simulink model "state_space_verification"  (R2023a)
settings: Solver=ode45  StartTime=0.0  StopTime=5  RelTol=1e-3
InitFcn:
  | data = load("state_space.mat");
  | A = data.A;
  | B = data.B;
  | 
  | K = test();
libraries: simulink_extras x8
settings Model: Creator=Jason  LastModifiedBy=Jason

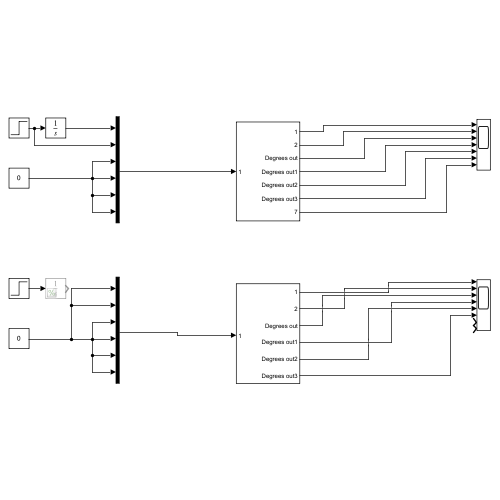
[thumbnail: Simulink's stored preview of the top-level diagram]
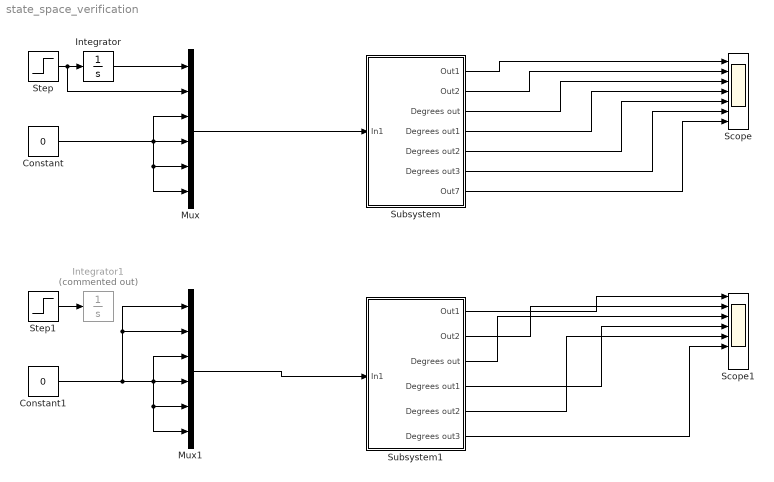
== system state_space_verification ==
  Constant : Constant  Value=0
  Constant1 : Constant  Value=0
  Integrator : Integrator
  Integrator1 : Integrator  Commented=on
  Mux : Mux  Inputs=6
  Mux1 : Mux  Inputs=6
  Scope : Scope  NumInputPorts=7
  Scope1 : Scope  NumInputPorts=8
  Step : Step  After=0.3  SampleTime=0
  Step1 : Step  SampleTime=0
  Subsystem : Subsystem
  Subsystem1 : Subsystem
  wires:
  Constant/1 -> Mux/3, Mux/6, Mux/5, Mux/4
  Step/1 -> Mux/2, Integrator/1
  Integrator/1 -> Mux/1
  Mux/1 -> Subsystem/1(In1)
  Subsystem/1(Out1) -> Scope/1
  Subsystem/2(Out2) -> Scope/2
  Subsystem/3(Degrees out) -> Scope/3
  Subsystem/4(Degrees out1) -> Scope/4
  Subsystem/5(Degrees out2) -> Scope/5
  Subsystem/6(Degrees out3) -> Scope/6
  Subsystem/7(Out7) -> Scope/7
  Constant1/1 -> Mux1/1, Mux1/2, Mux1/3, Mux1/6, Mux1/5, Mux1/4
  Step1/1 -> Integrator1/1
  Subsystem1/1(Out1) -> Scope1/1
  Subsystem1/3(Degrees out) -> Scope1/3
  Subsystem1/5(Degrees out2) -> Scope1/5
  Subsystem1/2(Out2) -> Scope1/2
  Subsystem1/4(Degrees out1) -> Scope1/4
  Subsystem1/6(Degrees out3) -> Scope1/6
  Mux1/1 -> Subsystem1/1(In1)

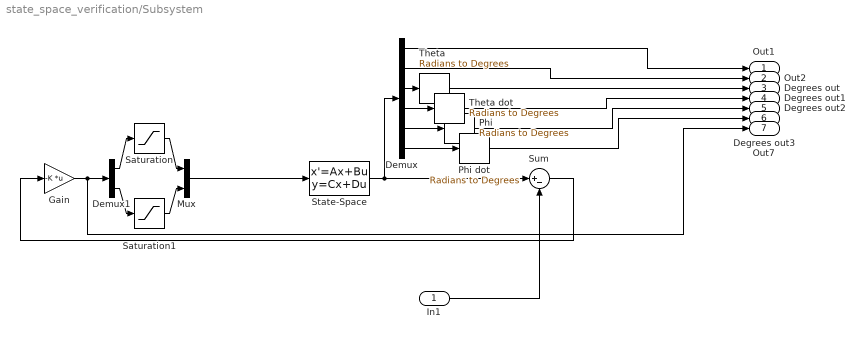
== system state_space_verification/Subsystem ==
  In1 : Inport
  Demux : Demux  Outputs=6
  Demux1 : Demux  Outputs=2
  Gain : Gain  Gain=-K  Multiplication=Matrix(K*u)
  Mux : Mux  Inputs=2
  Phi : simulink_extras/Transformations/Radians to Degrees
  Phi dot : simulink_extras/Transformations/Radians to Degrees
  Saturation : Saturate  UpperLimit=0.12  LowerLimit=-0.12
  Saturation1 : Saturate  UpperLimit=5  LowerLimit=-5
  State-Space : StateSpace  A=A  B=B  C=eye(6)  D=zeros(6,2)  InitialCondition=[0;0;0;0;0;0]
  Sum : Sum  Inputs=|+-
  Theta : simulink_extras/Transformations/Radians to Degrees
  Theta dot : simulink_extras/Transformations/Radians to Degrees
  Out1 : Outport
  Out2 : Outport  Port=2
  Degrees out : Outport  Port=3
  Degrees out1 : Outport  Port=4
  Degrees out2 : Outport  Port=5
  Degrees out3 : Outport  Port=6
  Out7 : Outport  Port=7
  wires:
  State-Space/1 -> Sum/1, Demux/1
  Demux/6 -> Phi dot/1
  Demux/3 -> Theta/1
  Phi/1 -> Degrees out2/1
  Sum/1 -> Gain/1
  Demux/5 -> Phi/1
  Demux/1 -> Out1/1
  Demux/4 -> Theta dot/1
  Theta/1 -> Degrees out/1
  Demux/2 -> Out2/1
  In1/1 -> Sum/2
  Theta dot/1 -> Degrees out1/1
  Phi dot/1 -> Degrees out3/1
  Gain/1 -> Out7/1, Demux1/1
  Demux1/2 -> Saturation1/1
  Demux1/1 -> Saturation/1
  Saturation/1 -> Mux/1
  Saturation1/1 -> Mux/2
  Mux/1 -> State-Space/1

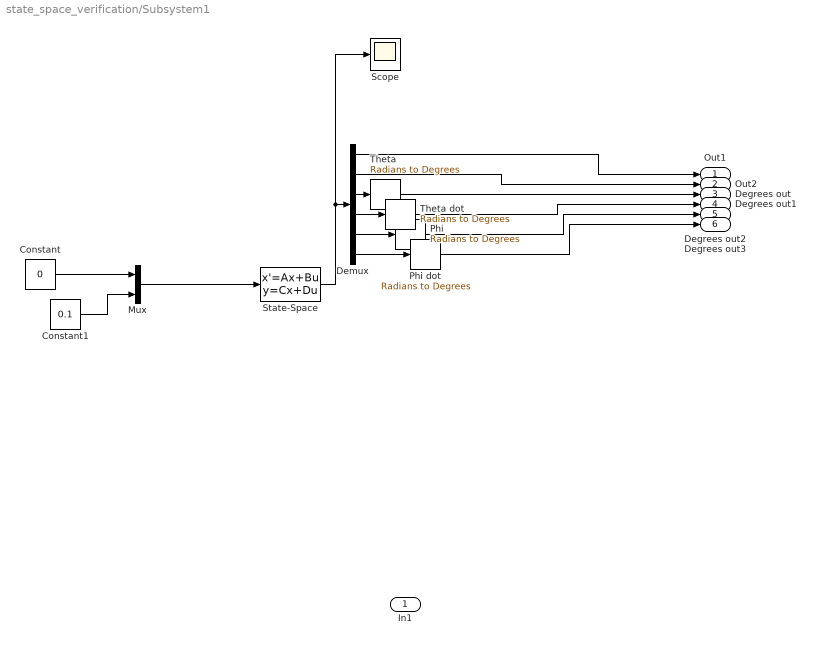
== system state_space_verification/Subsystem1 ==
  In1 : Inport
  Constant : Constant  Value=0
  Constant1 : Constant  Value=0.1
  Demux : Demux  Outputs=6
  Mux : Mux  Inputs=2
  Phi : simulink_extras/Transformations/Radians to Degrees
  Phi dot : simulink_extras/Transformations/Radians to Degrees
  Scope : Scope
  State-Space : StateSpace  A=A  B=B  C=eye(6)  D=zeros(6,2)  InitialCondition=[0;0;0.06981316889;0;0;0]
  Theta : simulink_extras/Transformations/Radians to Degrees
  Theta dot : simulink_extras/Transformations/Radians to Degrees
  Out1 : Outport
  Out2 : Outport  Port=2
  Degrees out : Outport  Port=3
  Degrees out1 : Outport  Port=4
  Degrees out2 : Outport  Port=5
  Degrees out3 : Outport  Port=6
  wires:
  State-Space/1 -> Scope/1, Demux/1
  Demux/6 -> Phi dot/1
  Demux/3 -> Theta/1
  Phi/1 -> Degrees out2/1
  Demux/5 -> Phi/1
  Demux/1 -> Out1/1
  Demux/4 -> Theta dot/1
  Theta/1 -> Degrees out/1
  Demux/2 -> Out2/1
  Theta dot/1 -> Degrees out1/1
  Phi dot/1 -> Degrees out3/1
  Mux/1 -> State-Space/1
  Constant/1 -> Mux/1
  Constant1/1 -> Mux/2
